simulink model "test_sim"  (R2015a)
settings: Solver=ode45  StartTime=0.0  StopTime=1  MaxStep=0.001  RelTol=1e-3
undefined symbols (not defined in the file or in its folder): carrier, F
settings Model: Creator=Karol  LastModifiedBy=Karol

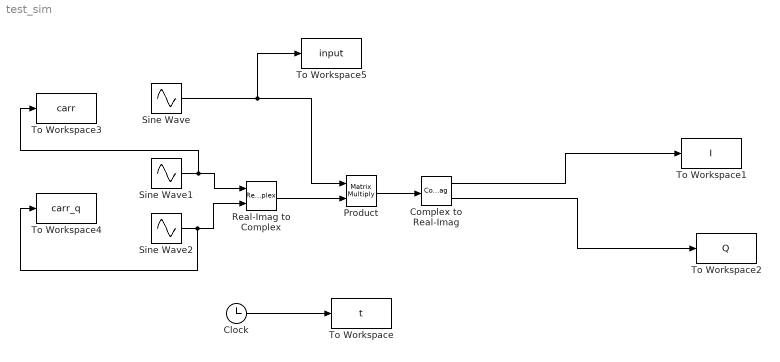
== system test_sim ==
  Clock : Clock
  Complex to Real-Imag : ComplexToRealImag
  Product : Product  Multiplication=Matrix(*)
  Real-Imag to Complex : RealImagToComplex
  Sine Wave : Sin  Frequency=F  SampleTime=0
  Sine Wave1 : Sin  Frequency=carrier  SampleTime=0
  Sine Wave2 : Sin  Frequency=carrier  Phase=-pi/2  SampleTime=0
  To Workspace : ToWorkspace  VariableName=t  SampleTime=-1
  To Workspace1 : ToWorkspace  VariableName=I  SampleTime=-1
  To Workspace2 : ToWorkspace  VariableName=Q  SampleTime=-1
  To Workspace3 : ToWorkspace  VariableName=carr  SampleTime=-1
  To Workspace4 : ToWorkspace  VariableName=carr_q  SampleTime=-1
  To Workspace5 : ToWorkspace  VariableName=input  SampleTime=-1
  wires:
  Clock/1 -> To Workspace/1
  Sine Wave1/1 -> To Workspace3/1, Real-Imag to Complex/1
  Sine Wave2/1 -> To Workspace4/1, Real-Imag to Complex/2
  Product/1 -> Complex to Real-Imag/1
  Sine Wave/1 -> Product/1, To Workspace5/1
  Real-Imag to Complex/1 -> Product/2
  Complex to Real-Imag/2 -> To Workspace2/1
  Complex to Real-Imag/1 -> To Workspace1/1
